simulink model "WaermepumpeGrundlage"  (R2013a)
settings: Solver=ode4  StartTime=0.0  StopTime=inf  RelTol=1e-3
libraries: Thermolib x73, simulink x2
(part 2 of 2)

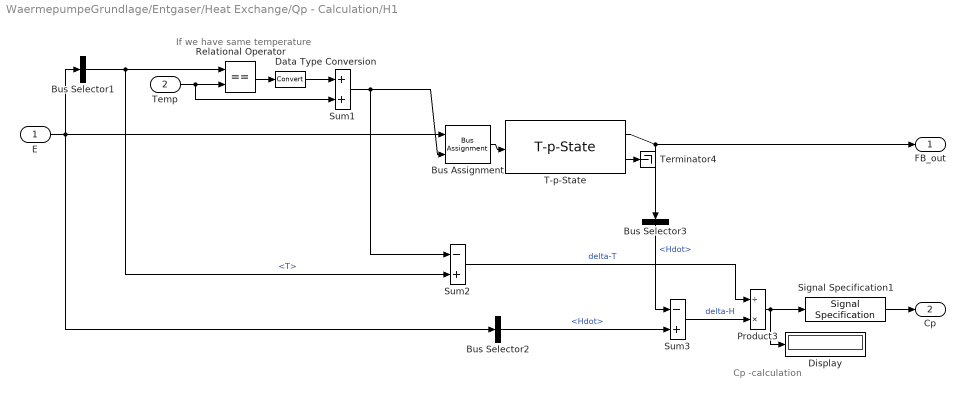
== system WaermepumpeGrundlage/Entgaser/Heat Exchange/Qp - Calculation/H1 ==
  note: Cp -calculation
  note: If we have same temperature
  E : Inport
  Temp : Inport  Port=2
  Bus Assignment : BusAssignment  AssignedSignals=T
  Bus Selector1 : BusSelector  OutputSignals=T
  Bus Selector2 : BusSelector  OutputSignals=Hdot
  Bus Selector3 : BusSelector  OutputSignals=Hdot
  Data Type Conversion : DataTypeConversion
  Display : Display
  Product3 : Product  Inputs=/*  SaturateOnIntegerOverflow=on  InputSameDT=on  OutDataTypeStr=Inherit: Same as first input
  Relational Operator : RelationalOperator  Operator===  OutDataTypeStr=boolean
  Signal Specification1 : SignalSpecification  Dimensions=1
  Sum1 : Sum  Inputs=2  SaturateOnIntegerOverflow=on  InputSameDT=on  OutDataTypeStr=Inherit: Same as first input
  Sum2 : Sum  Inputs=-+  SaturateOnIntegerOverflow=on  InputSameDT=on  OutDataTypeStr=Inherit: Same as first input
  Sum3 : Sum  Inputs=-+  SaturateOnIntegerOverflow=on  InputSameDT=on  OutDataTypeStr=Inherit: Same as first input
  T-p-State : Thermolib/Thermodynamic States and Properties/T-p-State
  Terminator4 : Terminator
  FB_out : Outport
  Cp : Outport  Port=2
  wires:
  T-p-State/2 -> Terminator4/1
  Sum1/1 -> Bus Assignment/2, Sum2/1
  Bus Selector1/1 -> Relational Operator/1, Sum2/2  "<T>"
  Bus Assignment/1 -> T-p-State/1
  T-p-State/1 -> FB_out/1, Bus Selector3/1
  E/1 -> Bus Selector1/1, Bus Selector2/1, Bus Assignment/1
  Temp/1 -> Relational Operator/2, Sum1/2
  Relational Operator/1 -> Data Type Conversion/1
  Data Type Conversion/1 -> Sum1/1
  Sum3/1 -> Product3/2  "delta-H"
  Sum2/1 -> Product3/1  "delta-T"
  Product3/1 -> Display/1, Signal Specification1/1
  Bus Selector2/1 -> Sum3/2  "<Hdot>"
  Bus Selector3/1 -> Sum3/1  "<Hdot>"
  Signal Specification1/1 -> Cp/1

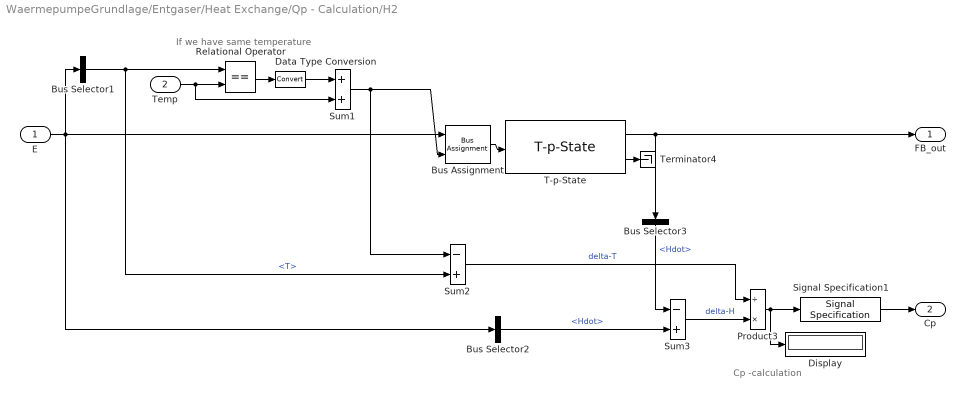
== system WaermepumpeGrundlage/Entgaser/Heat Exchange/Qp - Calculation/H2 ==
  note: If we have same temperature
  note: Cp -calculation
  E : Inport
  Temp : Inport  Port=2
  Bus Assignment : BusAssignment  AssignedSignals=T
  Bus Selector1 : BusSelector  OutputSignals=T
  Bus Selector2 : BusSelector  OutputSignals=Hdot
  Bus Selector3 : BusSelector  OutputSignals=Hdot
  Data Type Conversion : DataTypeConversion
  Display : Display
  Product3 : Product  Inputs=/*  SaturateOnIntegerOverflow=on  InputSameDT=on  OutDataTypeStr=Inherit: Same as first input
  Relational Operator : RelationalOperator  Operator===  OutDataTypeStr=boolean
  Signal Specification1 : SignalSpecification  Dimensions=1
  Sum1 : Sum  Inputs=2  SaturateOnIntegerOverflow=on  InputSameDT=on  OutDataTypeStr=Inherit: Same as first input
  Sum2 : Sum  Inputs=-+  SaturateOnIntegerOverflow=on  InputSameDT=on  OutDataTypeStr=Inherit: Same as first input
  Sum3 : Sum  Inputs=-+  SaturateOnIntegerOverflow=on  InputSameDT=on  OutDataTypeStr=Inherit: Same as first input
  T-p-State : Thermolib/Thermodynamic States and Properties/T-p-State
  Terminator4 : Terminator
  FB_out : Outport
  Cp : Outport  Port=2
  wires:
  T-p-State/2 -> Terminator4/1
  Bus Selector3/1 -> Sum3/1  "<Hdot>"
  Bus Selector2/1 -> Sum3/2  "<Hdot>"
  Product3/1 -> Display/1, Signal Specification1/1
  Sum2/1 -> Product3/1  "delta-T"
  Sum3/1 -> Product3/2  "delta-H"
  Data Type Conversion/1 -> Sum1/1
  Relational Operator/1 -> Data Type Conversion/1
  Temp/1 -> Sum1/2, Relational Operator/2
  E/1 -> Bus Assignment/1, Bus Selector2/1, Bus Selector1/1
  T-p-State/1 -> Bus Selector3/1, FB_out/1
  Bus Assignment/1 -> T-p-State/1
  Bus Selector1/1 -> Sum2/2, Relational Operator/1  "<T>"
  Sum1/1 -> Sum2/1, Bus Assignment/2
  Signal Specification1/1 -> Cp/1

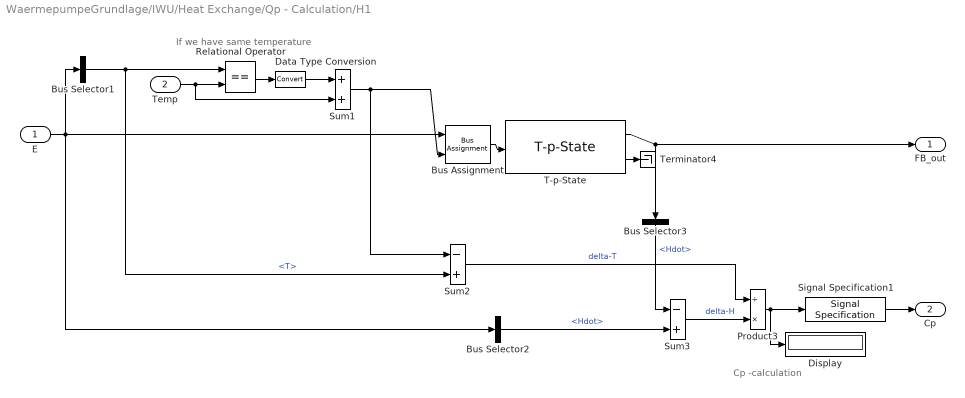
== system WaermepumpeGrundlage/IWU/Heat Exchange/Qp - Calculation/H1 ==
  note: If we have same temperature
  note: Cp -calculation
  E : Inport
  Temp : Inport  Port=2
  Bus Assignment : BusAssignment  AssignedSignals=T
  Bus Selector1 : BusSelector  OutputSignals=T
  Bus Selector2 : BusSelector  OutputSignals=Hdot
  Bus Selector3 : BusSelector  OutputSignals=Hdot
  Data Type Conversion : DataTypeConversion
  Display : Display
  Product3 : Product  Inputs=/*  SaturateOnIntegerOverflow=on  InputSameDT=on  OutDataTypeStr=Inherit: Same as first input
  Relational Operator : RelationalOperator  Operator===  OutDataTypeStr=boolean
  Signal Specification1 : SignalSpecification  Dimensions=1
  Sum1 : Sum  Inputs=2  SaturateOnIntegerOverflow=on  InputSameDT=on  OutDataTypeStr=Inherit: Same as first input
  Sum2 : Sum  Inputs=-+  SaturateOnIntegerOverflow=on  InputSameDT=on  OutDataTypeStr=Inherit: Same as first input
  Sum3 : Sum  Inputs=-+  SaturateOnIntegerOverflow=on  InputSameDT=on  OutDataTypeStr=Inherit: Same as first input
  T-p-State : Thermolib/Thermodynamic States and Properties/T-p-State
  Terminator4 : Terminator
  FB_out : Outport
  Cp : Outport  Port=2
  wires:
  Signal Specification1/1 -> Cp/1
  Bus Selector3/1 -> Sum3/1  "<Hdot>"
  Bus Selector2/1 -> Sum3/2  "<Hdot>"
  Product3/1 -> Signal Specification1/1, Display/1
  Sum2/1 -> Product3/1  "delta-T"
  Sum3/1 -> Product3/2  "delta-H"
  Data Type Conversion/1 -> Sum1/1
  Relational Operator/1 -> Data Type Conversion/1
  Temp/1 -> Sum1/2, Relational Operator/2
  E/1 -> Bus Assignment/1, Bus Selector2/1, Bus Selector1/1
  T-p-State/1 -> Bus Selector3/1, FB_out/1
  Bus Assignment/1 -> T-p-State/1
  Bus Selector1/1 -> Sum2/2, Relational Operator/1  "<T>"
  Sum1/1 -> Sum2/1, Bus Assignment/2
  T-p-State/2 -> Terminator4/1

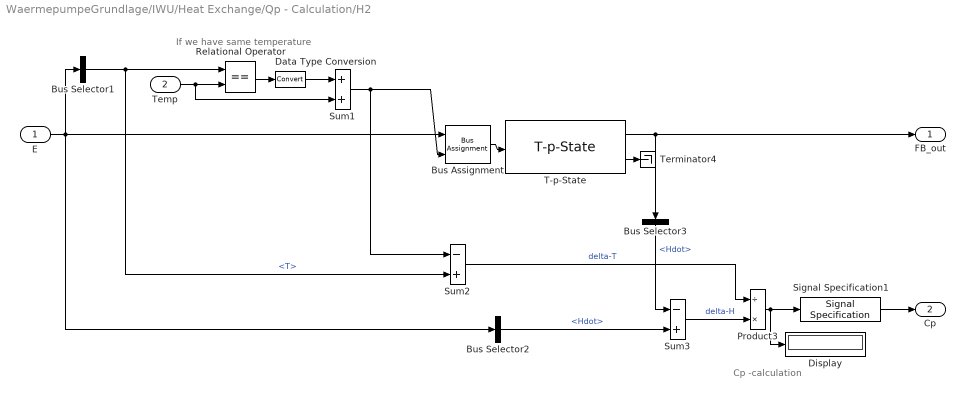
== system WaermepumpeGrundlage/IWU/Heat Exchange/Qp - Calculation/H2 ==
  note: Cp -calculation
  note: If we have same temperature
  E : Inport
  Temp : Inport  Port=2
  Bus Assignment : BusAssignment  AssignedSignals=T
  Bus Selector1 : BusSelector  OutputSignals=T
  Bus Selector2 : BusSelector  OutputSignals=Hdot
  Bus Selector3 : BusSelector  OutputSignals=Hdot
  Data Type Conversion : DataTypeConversion
  Display : Display
  Product3 : Product  Inputs=/*  SaturateOnIntegerOverflow=on  InputSameDT=on  OutDataTypeStr=Inherit: Same as first input
  Relational Operator : RelationalOperator  Operator===  OutDataTypeStr=boolean
  Signal Specification1 : SignalSpecification  Dimensions=1
  Sum1 : Sum  Inputs=2  SaturateOnIntegerOverflow=on  InputSameDT=on  OutDataTypeStr=Inherit: Same as first input
  Sum2 : Sum  Inputs=-+  SaturateOnIntegerOverflow=on  InputSameDT=on  OutDataTypeStr=Inherit: Same as first input
  Sum3 : Sum  Inputs=-+  SaturateOnIntegerOverflow=on  InputSameDT=on  OutDataTypeStr=Inherit: Same as first input
  T-p-State : Thermolib/Thermodynamic States and Properties/T-p-State
  Terminator4 : Terminator
  FB_out : Outport
  Cp : Outport  Port=2
  wires:
  Signal Specification1/1 -> Cp/1
  Sum1/1 -> Bus Assignment/2, Sum2/1
  Bus Selector1/1 -> Relational Operator/1, Sum2/2  "<T>"
  Bus Assignment/1 -> T-p-State/1
  T-p-State/1 -> FB_out/1, Bus Selector3/1
  E/1 -> Bus Selector1/1, Bus Selector2/1, Bus Assignment/1
  Temp/1 -> Relational Operator/2, Sum1/2
  Relational Operator/1 -> Data Type Conversion/1
  Data Type Conversion/1 -> Sum1/1
  Sum3/1 -> Product3/2  "delta-H"
  Sum2/1 -> Product3/1  "delta-T"
  Product3/1 -> Signal Specification1/1, Display/1
  Bus Selector2/1 -> Sum3/2  "<Hdot>"
  Bus Selector3/1 -> Sum3/1  "<Hdot>"
  T-p-State/2 -> Terminator4/1
